simulink model "Lab3"  (R2024b)
settings: Solver=VariableStepAuto  StartTime=0.0  StopTime=.04  RelTol=1e-3
libraries: spsRMSLib x4, spsSeriesRLCLoadLib x2, spsCurrentMeasurementLib x2, eePowerMeasurement x2, spsVoltageMeasurementLib x2, spsACVoltageSourceLib x1, spsSeriesRLCBranchLib x1, sps_lib x1
settings Model: Creator=Jamil!  LastModifiedBy=Jamil!

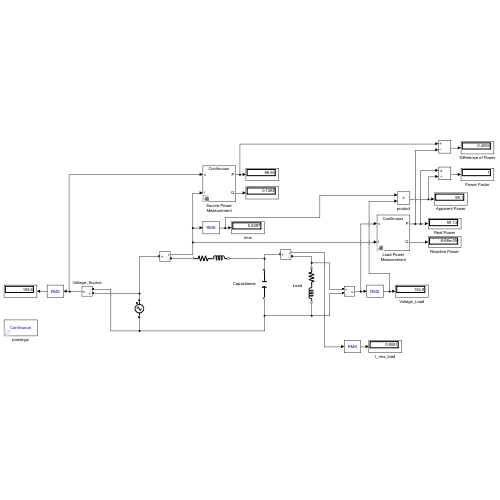
[thumbnail: Simulink's stored preview of the top-level diagram]
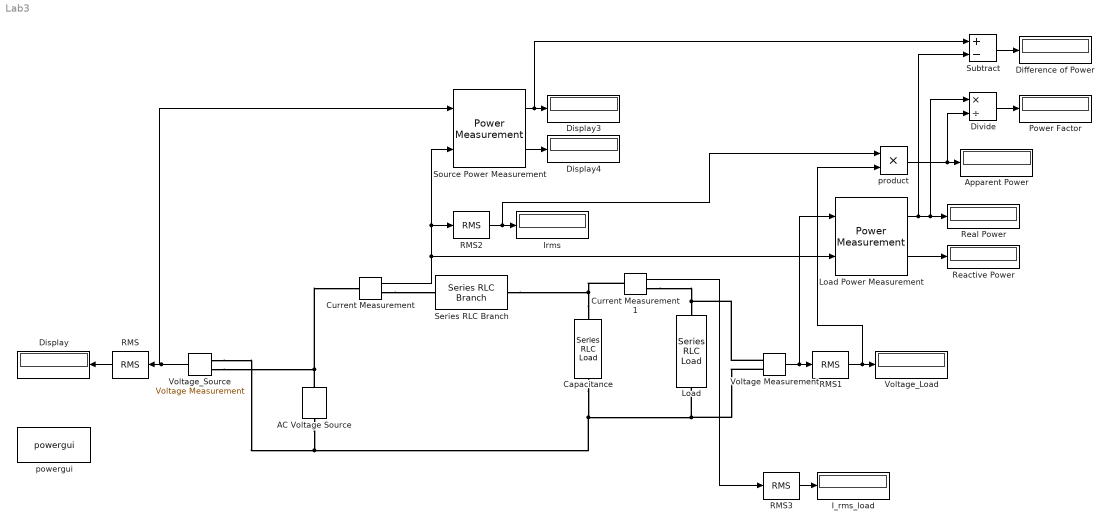
== system Lab3 ==
  AC Voltage Source : spsACVoltageSourceLib/AC Voltage Source  Amplitude=220  Phase=0  Frequency=50  SampleTime=0  Measurements=None  BusType=swing  Pref=10e3  Qref=0  Qmin=-inf  Qmax=+inf
  Apparent Power : Display
  Capacitance : spsSeriesRLCLoadLib/Series RLC Load  LConnTagsString=a  RConnTagsString=__new0  NominalVoltage=155.6  NominalFrequency=50  ActivePower=0  InductivePower=0  CapacitivePower=100  Setx0=off  InitialVoltage=0  SetiL0=off  InitialCurrent=0  Measurements=None  LoadType=constant Z
  Current Measurement : spsCurrentMeasurementLib/Current Measurement  PhasorSimulation=off  OutputType=Complex  PSBequivalent=0
  Current Measurement1 : spsCurrentMeasurementLib/Current Measurement  PhasorSimulation=off  OutputType=Complex  PSBequivalent=0
  Difference of Power : Display
  Display : Display
  Display3 : Display
  Display4 : Display
  Divide : Product  Inputs=*/
  I_rms_load : Display
  Irms : Display
  Load : spsSeriesRLCLoadLib/Series RLC Load  LConnTagsString=a  RConnTagsString=__new0  NominalVoltage=155.6  NominalFrequency=50  ActivePower=100  InductivePower=100  CapacitivePower=0  Setx0=off  InitialVoltage=0  SetiL0=off  InitialCurrent=0  Measurements=None  LoadType=constant Z
  Load Power Measurement : eePowerMeasurement/Power Measurement  LabelModeActiveChoice=Continuous  F=50  K=[1]  Ts=0
  Power Factor : Display
  RMS{,1..3} (4 alike) : spsRMSLib/RMS  TrueRMS=on  Freq=50  RMSInit=120  Ts=0
  Reactive Power : Display
  Real Power : Display
  Series RLC Branch : spsSeriesRLCBranchLib/Series RLC Branch  LConnTagsString=__new0  RConnTagsString=__new0  BranchType=RL  Resistance=1  Inductance=0.001  SetiL0=off  InitialCurrent=0  Capacitance=1e-6  Setx0=off  InitialVoltage=0  Measurements=None
  Source Power Measurement : eePowerMeasurement/Power Measurement  LabelModeActiveChoice=Continuous  F=50  K=[1]  Ts=0
  Subtract : Sum  Inputs=+-
  Voltage Measurement : spsVoltageMeasurementLib/Voltage Measurement  PhasorSimulation=off  OutputType=Complex  PSBequivalent=0
  Voltage_Load : Display
  Voltage_Source : spsVoltageMeasurementLib/Voltage Measurement  PhasorSimulation=off  OutputType=Complex  PSBequivalent=0
  powergui : sps_lib/powergui  Priority=1  SimulationMode=Continuous  SampleTime=50e-6  frequency=60  Iterations=50  frequencyindice=50  Pbase=100e6  ErrMax=1e-4  UnitsV=kV  UnitsW=MW  buscounter=0  FunctionMessages=off  echomessages=off  EnableUseOfTLC=off  CurrentSourceSwitches=off  DisableSnubberDevices=off  DisableRonSwitches=off  DisableVfSwitches=off  DisplayEquations=off  AutomaticDiscreteSolvers=off  SolverType=Tustin/Backward Euler (TBE)  Interpol=off  ExternalGateDelay=off  methode=off  Ts=100  x0status=blocks  SPID=on  SwTol=0  HookPort=off  NonlinearTolerance=1e-4  nMaxIteration=100  ContinueOnMaxIteration=off  RestoreLinks=warning  ResistiveCurrentMeasurement=off  Frange=[0:2:500]  Ylog=off  Xlog=on  ShowGrid=off  save=off  variable=ZData  structure=0  ZoomFFT=off  StartTime=0.0  cycles=1  DisplayStyle=1  fundamental=60  FreqAxis=off  MaxFrequency=1000  frequencyindicesteady=1  RmsSteady=1  display=off
  product : Product
  wires:
  Voltage_Source/1 -> Source Power Measurement/1, RMS/1
  Current Measurement/1 -> Load Power Measurement/2, RMS2/1, Source Power Measurement/2
  Load Power Measurement/2 -> Reactive Power/1
  Subtract/1 -> Difference of Power/1
  product/1 -> Divide/2, Apparent Power/1
  RMS3/1 -> I_rms_load/1
  Source Power Measurement/1 -> Subtract/1, Display3/1
  Current Measurement1/1 -> RMS3/1
  RMS2/1 -> product/1, Irms/1
  Voltage Measurement/1 -> Load Power Measurement/1, RMS1/1
  Source Power Measurement/2 -> Display4/1
  RMS1/1 -> product/2, Voltage_Load/1
  RMS/1 -> Display/1
  Divide/1 -> Power Factor/1
  Load Power Measurement/1 -> Subtract/2, Divide/1, Real Power/1
  connections:
  Load/LConn1 -- Voltage Measurement/LConn1 -- Current Measurement1/RConn1
  Load/RConn1 -- AC Voltage Source/LConn1 -- Voltage_Source/LConn2 -- Capacitance/RConn1 -- Voltage Measurement/LConn2
  Voltage_Source/LConn1 -- Current Measurement/LConn1 -- AC Voltage Source/RConn1
  Capacitance/LConn1 -- Current Measurement1/LConn1 -- Series RLC Branch/RConn1
  Current Measurement/RConn1 -- Series RLC Branch/LConn1
